simulink model "Testing_Serial_Comm"  (R2022a)
settings: Solver=FixedStepAuto  StartTime=0.0  StopTime=100.0  FixedStep=1e-3  RelTol=1e-3  EnableMultiTasking=on
libraries: frdmk64flib x3
settings Model: ExtModeTrigDuration=5  Creator=ethan  LastModifiedBy=ethan
settings OptimizationCC: EnhancedBackFolding=on  PassReuseOutputArgsAs=Individual arguments  ZeroExternalMemoryAtStartup=off  ZeroInternalMemoryAtStartup=off  MaxStackSize=64  OptimizeBlockOrder=speed  DifferentSizesBufferReuse=on  OptimizationCustomize=off  EfficientTunableParamExpr=on
settings DebuggingCC: ParameterTunabilityLossMsg=error
settings HardwareCC: ProdBitPerPointer=32  ProdBitPerSizeT=32  ProdBitPerPtrDiffT=32  ProdLargestAtomicInteger=Long  ProdLargestAtomicFloat=Double  ProdWordSize=32  ProdHWDeviceType=ARM Compatible->ARM Cortex
settings SFSimCC: MATLABDynamicMemAlloc=off
settings RTWCC: SystemTargetFile=ert.tlc  HardwareBoard=NXP FRDM-K64F  TLCOptions="-aInlineSetEventsForThisBaseRateFcn=TLC_FALSE -aSuppressMultiTaskScheduler=TLC_FALSE  -aRateBasedStepFcn=0"  TemplateMakefile=ert_default_tmf  Toolchain=GNU Tools for ARM Embedded Processors
settings CodeAppCC: ForceParamTrailComments=on  IgnoreCustomStorageClasses=off  OperatorAnnotations=on  SimulinkDataObjDesc=on  SFDataObjDesc=on  InsertBlockDesc=on
settings ERTTargetCC: ExtModeTransport=4  ExtModeMexFile=sendToCommService

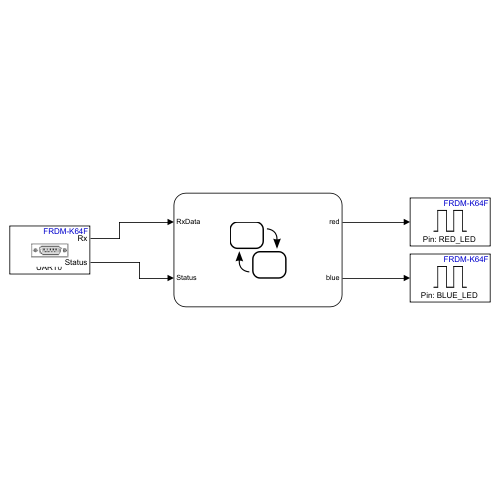
[thumbnail: Simulink's stored preview of the top-level diagram]
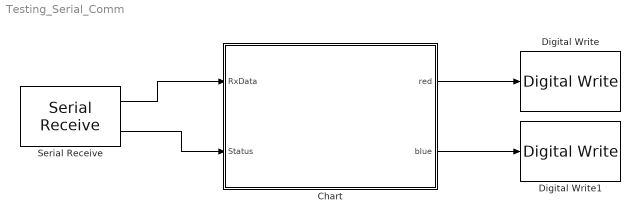
== system Testing_Serial_Comm ==
  Chart : Stateflow chart  TreatAsAtomicUnit=on
  Digital Write : frdmk64flib/Digital Write  Whichpin=RED_LED
  Digital Write1 : frdmk64flib/Digital Write  Whichpin=BLUE_LED
  Serial Receive : frdmk64flib/Serial Receive  SCIModule=0  Baudrate=uint32(9600)  Parity=None  StopBits=1  HardwareFlowControl=None  ByteOrder=LittleEndian  DataType=uint8  DataLength=2  BlockingMode=off  OutputStatus=on  SampleTime=-1
  wires:
  Serial Receive/1 -> Chart/1(RxData)
  Chart/1(red) -> Digital Write/1
  Chart/2(blue) -> Digital Write1/1
  Serial Receive/2 -> Chart/2(Status)

== stateflow chart Testing_Serial_Comm/Chart ==
  settings: executeAtInitialization=1
  state Data_Recieved1
    entry:
    red = false;
    blue = true;
  state Initialize_Variables
    entry:
    red = false;
    blue = false;
  state Data_Not_Recieved
  state Data_Recieved
    entry:
    red = true;
    blue = false;
  Data_Recieved1 -> Initialize_Variables : after(500,msec)
  (junction 25) -> Data_Recieved1 [order 2] : [RxData(2) == hex2dec('20')]
  (junction 18) -> Data_Not_Recieved [order 2]
  (default) -> Initialize_Variables
  Data_Not_Recieved -> (junction 18) : [Status == 0]
  (junction 18) -> (junction 25) [order 1] : [RxData(1) == hex2dec('10')]
  Initialize_Variables -> Data_Not_Recieved
  (junction 25) -> Data_Recieved [order 1] : [RxData(2) == hex2dec('30')]
  Data_Recieved -> Initialize_Variables : after(500,msec)
  data: RxData input; Status input; red output; blue output
